simulink model "nn_fuel_control_5_10"  (R2021a)
settings: Solver=ode15s  StartTime=0.0  StopTime=T  MaxStep=.01  RelTol=1e-3
undefined symbols (not defined in the file): AF_sensor_tol, fault_time, fuel_inj_tol, kappa_tol, MAF_sensor_tol, pump_tol, tau_ww_tol
libraries: neural x57
(part 2 of 2)

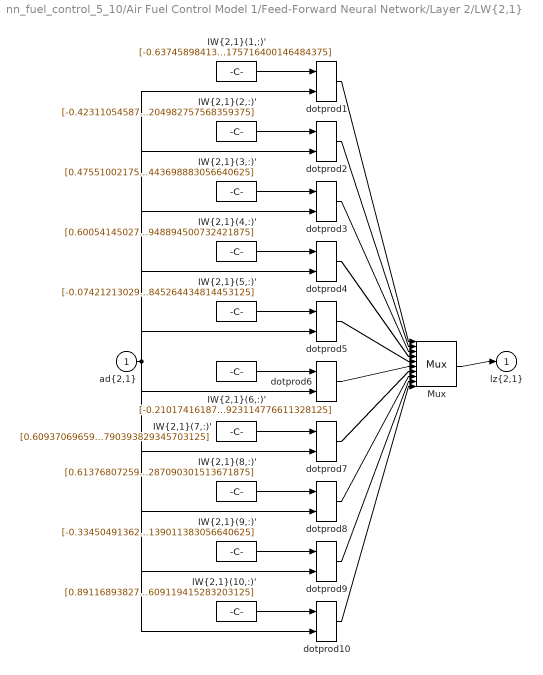
== system nn_fuel_control_5_10/Air Fuel Control Model 1/Feed-Forward Neural Network/Layer 2/LW{2,1} ==
  "ad{2,1}" : Inport  PortDimensions=10
      mask Display: e = 0.06;c1 = [120 230 180]/255;c2 = ([120 230 180]+0)/(256+128);c3 = ([120 230 180]+128)/(256+128);patch([0 1 1 0],[0 0 1 1],c1);patch([0 1 1 1-e 1-e 0+e],[0 0 1 1-e 0+e 0+e],c2);patch([0 0 1 1-e 0+e 0+e],[0 1 1 1-e 1-e 0+e],c3);plot([0 1 1 0 0],[0 0 1 1 0]);
  "IW{2,1}(1,:)'" : Constant  Value=[-0.637458984139413598057899434934370219707489013671875;0.8966217246671168705773879992193542420864105224609375;-0.0203090886026930927954481376218609511852264404296875;-0.412824398884275911569829986547119915485382080078125;-0.2423503469494130424521927125169895589351654052734375;0.9041152712576534522526117143570445477962493896484375;0.0771360103896812088208889690577052533626556396484375;-0.5024621550745056453024517395533621311187744140625;-0.2575893308760581756899910033098421990871429443359375;-0.6905985775161285200596239519654773175716400146484375]
      mask Display: e = 0.06;c1 = [120 150 230]/255;c2 = ([120 150 230]+0)/383;c3 = ([120 150 230]+128)/383;patch([0 1 1 0],[0 0 1 1],c1);patch([0 1 1 1-e 1-e 0+e],[0 0 1 1-e 0+e 0+e],c2);patch([0 0 1 1-e 0+e 0+e],[0 1 1 1-e 1-e 0+e],c3);plot([0 1 1 0 0],[0 0 1 1 0]);disp('weights');
  "IW{2,1}(10,:)'" : Constant  Value=[0.89116893827174614717279155229334719479084014892578125;-0.138771685053732329873099615724640898406505584716796875;0.360066357677085335797784182432224042713642120361328125;-0.486266631272339822089634253643453121185302734375;0.70490108854026178875074037932790815830230712890625;-0.96673858598125861352201582121779210865497589111328125;-0.206458691092018031820742862691986374557018280029296875;-0.96339598717867447330576169406413100659847259521484375;0.8351387726501771080478420117287896573543548583984375;0.2185868428207282665454158632201142609119415283203125]
      mask Display: e = 0.06;c1 = [120 150 230]/255;c2 = ([120 150 230]+0)/383;c3 = ([120 150 230]+128)/383;patch([0 1 1 0],[0 0 1 1],c1);patch([0 1 1 1-e 1-e 0+e],[0 0 1 1-e 0+e 0+e],c2);patch([0 0 1 1-e 0+e 0+e],[0 1 1 1-e 1-e 0+e],c3);plot([0 1 1 0 0],[0 0 1 1 0]);disp('weights');
  "IW{2,1}(2,:)'" : Constant  Value=[-0.423110545874279708744580830170889385044574737548828125;0.2368532384729105377818569877490517683327198028564453125;1.0125614808797680499452553704031743109226226806640625;0.991350908230053118330715733463875949382781982421875;0.5859879599201758271220796814304776489734649658203125;0.6228416385910036101591913393349386751651763916015625;0.66297446165075479829198457082384265959262847900390625;-0.68249454455804670072183171214419417083263397216796875;-0.2731411644690309170613318201503716409206390380859375;0.7259508101752485398350245304754935204982757568359375]
      mask Display: e = 0.06;c1 = [120 150 230]/255;c2 = ([120 150 230]+0)/383;c3 = ([120 150 230]+128)/383;patch([0 1 1 0],[0 0 1 1],c1);patch([0 1 1 1-e 1-e 0+e],[0 0 1 1-e 0+e 0+e],c2);patch([0 0 1 1-e 0+e 0+e],[0 1 1 1-e 1-e 0+e],c3);plot([0 1 1 0 0],[0 0 1 1 0]);disp('weights');
  "IW{2,1}(3,:)'" : Constant  Value=[0.47551002175782264291825640611932612955570220947265625;0.08086399994805872071257368816077359952032566070556640625;0.65153887054984982452054964596754871308803558349609375;-0.390853469357781424520226210006512701511383056640625;0.4244387850223023672668887229519896209239959716796875;0.69780646247800970360941619219374842941761016845703125;-0.422605255513745337037079252695548348128795623779296875;0.1356374397477954907298425268891151063144207000732421875;-0.799602102088680322111713394406251609325408935546875;0.3829313320921274854669036358245648443698883056640625]
      mask Display: e = 0.06;c1 = [120 150 230]/255;c2 = ([120 150 230]+0)/383;c3 = ([120 150 230]+128)/383;patch([0 1 1 0],[0 0 1 1],c1);patch([0 1 1 1-e 1-e 0+e],[0 0 1 1-e 0+e 0+e],c2);patch([0 0 1 1-e 0+e 0+e],[0 1 1 1-e 1-e 0+e],c3);plot([0 1 1 0 0],[0 0 1 1 0]);disp('weights');
  "IW{2,1}(4,:)'" : Constant  Value=[0.6005414502795767273113369810744188725948333740234375;11.4320674147867809011813733377493917942047119140625;0.421951948405398014063649725358118303120136260986328125;-0.037861256050832903241598614840768277645111083984375;-0.9949671896674103788171805717865936458110809326171875;-0.199969021175616656904594492516480386257171630859375;0.935316259593251597692642462789081037044525146484375;-0.94904454226816470363559119505225680768489837646484375;0.85670612621257102858862708671949803829193115234375;0.0801975162350963000079673292930237948894500732421875]
      mask Display: e = 0.06;c1 = [120 150 230]/255;c2 = ([120 150 230]+0)/383;c3 = ([120 150 230]+128)/383;patch([0 1 1 0],[0 0 1 1],c1);patch([0 1 1 1-e 1-e 0+e],[0 0 1 1-e 0+e 0+e],c2);patch([0 0 1 1-e 0+e 0+e],[0 1 1 1-e 1-e 0+e],c3);plot([0 1 1 0 0],[0 0 1 1 0]);disp('weights');
  "IW{2,1}(5,:)'" : Constant  Value=[-0.0742121302954270589680163539014756679534912109375;-0.1342580978786223067089622418279759585857391357421875;0.0915832479993226034054032425046898424625396728515625;-0.93787302986105913760184193961322307586669921875;-0.643811203007536025921808686689473688602447509765625;-0.116756066682536019385452163987793028354644775390625;-0.1435483736603855309255095562548376619815826416015625;-0.5110511184347534818783742593950591981410980224609375;-0.758544811567411603192567781661637127399444580078125;-0.398523306888638462197604894754476845264434814453125]
      mask Display: e = 0.06;c1 = [120 150 230]/255;c2 = ([120 150 230]+0)/383;c3 = ([120 150 230]+128)/383;patch([0 1 1 0],[0 0 1 1],c1);patch([0 1 1 1-e 1-e 0+e],[0 0 1 1-e 0+e 0+e],c2);patch([0 0 1 1-e 0+e 0+e],[0 1 1 1-e 1-e 0+e],c3);plot([0 1 1 0 0],[0 0 1 1 0]);disp('weights');
  "IW{2,1}(6,:)'" : Constant  Value=[-0.210174161874227660717906474019400775432586669921875;-0.3228525547071037227198075925116427242755889892578125;0.081467094240803117344285055878572165966033935546875;-0.223563749699733360642994739464484155178070068359375;0.55022795910762933857540701865218579769134521484375;0.1733910151474036265284439650713466107845306396484375;-0.4722076811425550690870522885234095156192779541015625;-0.7008127640379659961666902745491825044155120849609375;-0.7519677194670675302035078857443295419216156005859375;-0.134393425407410394001317399670369923114776611328125]
      mask Display: e = 0.06;c1 = [120 150 230]/255;c2 = ([120 150 230]+0)/383;c3 = ([120 150 230]+128)/383;patch([0 1 1 0],[0 0 1 1],c1);patch([0 1 1 1-e 1-e 0+e],[0 0 1 1-e 0+e 0+e],c2);patch([0 0 1 1-e 0+e 0+e],[0 1 1 1-e 1-e 0+e],c3);plot([0 1 1 0 0],[0 0 1 1 0]);disp('weights');
  "IW{2,1}(7,:)'" : Constant  Value=[0.6093706965999181601745249281520955264568328857421875;0.3953690665368394530077011950197629630565643310546875;0.084179609944530164877818378954543732106685638427734375;0.4749507737805398477348717278800904750823974609375;0.66685673515731735960798687301576137542724609375;0.478883610897159084363039482923340983688831329345703125;-0.1708217128254700956091483021737076342105865478515625;0.268209410222957078673289288417436182498931884765625;-0.97388905831939087676119015668518841266632080078125;-0.4246705658523748372346062751603312790393829345703125]
      mask Display: e = 0.06;c1 = [120 150 230]/255;c2 = ([120 150 230]+0)/383;c3 = ([120 150 230]+128)/383;patch([0 1 1 0],[0 0 1 1],c1);patch([0 1 1 1-e 1-e 0+e],[0 0 1 1-e 0+e 0+e],c2);patch([0 0 1 1-e 0+e 0+e],[0 1 1 1-e 1-e 0+e],c3);plot([0 1 1 0 0],[0 0 1 1 0]);disp('weights');
  "IW{2,1}(8,:)'" : Constant  Value=[0.6137680725996259578636227161041460931301116943359375;-1.191467660059975397501830229884944856166839599609375;0.7756199138359132216891111966106109321117401123046875;-0.837639262904835479872645009891130030155181884765625;0.89500835157132652142308870679698884487152099609375;-0.45248395209114200543609740634565241634845733642578125;0.241077681509801300396844681017682887613773345947265625;0.234555770444050681877712349887588061392307281494140625;-0.7503101997745991180721603086567483842372894287109375;0.690380892111544852696169982664287090301513671875]
      mask Display: e = 0.06;c1 = [120 150 230]/255;c2 = ([120 150 230]+0)/383;c3 = ([120 150 230]+128)/383;patch([0 1 1 0],[0 0 1 1],c1);patch([0 1 1 1-e 1-e 0+e],[0 0 1 1-e 0+e 0+e],c2);patch([0 0 1 1-e 0+e 0+e],[0 1 1 1-e 1-e 0+e],c3);plot([0 1 1 0 0],[0 0 1 1 0]);disp('weights');
  "IW{2,1}(9,:)'" : Constant  Value=[-0.3345049136284374835526023161946795880794525146484375;0.18594208697542580210892992909066379070281982421875;0.6455995939500607239125429259729571640491485595703125;-0.7707899293641851112823815128649584949016571044921875;-0.075594471798157147901520147570408880710601806640625;0.06163623848505039859446696937084197998046875;-0.213693913452614570047671804786659777164459228515625;-0.6393005766123474042927909977152012288570404052734375;-0.6056315881196070449732360430061817169189453125;-0.2241069216575370948163481443771161139011383056640625]
      mask Display: e = 0.06;c1 = [120 150 230]/255;c2 = ([120 150 230]+0)/383;c3 = ([120 150 230]+128)/383;patch([0 1 1 0],[0 0 1 1],c1);patch([0 1 1 1-e 1-e 0+e],[0 0 1 1-e 0+e 0+e],c2);patch([0 0 1 1-e 0+e 0+e],[0 1 1 1-e 1-e 0+e],c3);plot([0 1 1 0 0],[0 0 1 1 0]);disp('weights');
  Mux : Mux  Inputs=10
      mask Display: e = 0.06;c1 = [120 150 230]/255;c2 = ([120 150 230]+0)/383;c3 = ([120 150 230]+128)/383;patch([0 1 1 0],[0 0 1 1],c1);patch([0 1 1 1-e 1-e 0+e],[0 0 1 1-e 0+e 0+e],c2);patch([0 0 1 1-e 0+e 0+e],[0 1 1 1-e 1-e 0+e],c3);plot([0 1 1 0 0],[0 0 1 1 0]);disp('Mux');
  dotprod{1..10} (10 alike) : neural/Weight Functions/dotprod
  "lz{2,1}" : Outport
      mask Display: e = 0.06;c1 = [120 230 180]/255;c2 = ([120 230 180]+0)/(256+128);c3 = ([120 230 180]+128)/(256+128);patch([0 1 1 0],[0 0 1 1],c1);patch([0 1 1 1-e 1-e 0+e],[0 0 1 1-e 0+e 0+e],c2);patch([0 0 1 1-e 0+e 0+e],[0 1 1 1-e 1-e 0+e],c3);plot([0 1 1 0 0],[0 0 1 1 0]);
  wires:
  "IW{2,1}(1,:)'"/1 -> dotprod1/1
  "ad{2,1}"/1 -> dotprod1/2, dotprod2/2, dotprod3/2, dotprod4/2, dotprod5/2, dotprod6/2, dotprod7/2, dotprod8/2, dotprod9/2, dotprod10/2
  dotprod1/1 -> Mux/1
  "IW{2,1}(2,:)'"/1 -> dotprod2/1
  dotprod2/1 -> Mux/2
  "IW{2,1}(3,:)'"/1 -> dotprod3/1
  dotprod3/1 -> Mux/3
  "IW{2,1}(4,:)'"/1 -> dotprod4/1
  dotprod4/1 -> Mux/4
  "IW{2,1}(5,:)'"/1 -> dotprod5/1
  dotprod5/1 -> Mux/5
  "IW{2,1}(6,:)'"/1 -> dotprod6/1
  dotprod6/1 -> Mux/6
  "IW{2,1}(7,:)'"/1 -> dotprod7/1
  dotprod7/1 -> Mux/7
  "IW{2,1}(8,:)'"/1 -> dotprod8/1
  dotprod8/1 -> Mux/8
  "IW{2,1}(9,:)'"/1 -> dotprod9/1
  dotprod9/1 -> Mux/9
  "IW{2,1}(10,:)'"/1 -> dotprod10/1
  dotprod10/1 -> Mux/10
  Mux/1 -> "lz{2,1}"/1

== system nn_fuel_control_5_10/Air Fuel Control Model 1/Feed-Forward Neural Network/Layer 3/Delays 1 ==
  "p{3}" : Inport  PortDimensions=10
      mask Display: e = 0.06;c1 = [120 230 180]/255;c2 = ([120 230 180]+0)/(256+128);c3 = ([120 230 180]+128)/(256+128);patch([0 1 1 0],[0 0 1 1],c1);patch([0 1 1 1-e 1-e 0+e],[0 0 1 1-e 0+e 0+e],c2);patch([0 0 1 1-e 0+e 0+e],[0 1 1 1-e 1-e 0+e],c3);plot([0 1 1 0 0],[0 0 1 1 0]);
  mux : Mux  Inputs=1
      mask Display: e = 0.06;c1 = [120 150 230]/255;c2 = ([120 150 230]+0)/383;c3 = ([120 150 230]+128)/383;patch([0 1 1 0],[0 0 1 1],c1);patch([0 1 1 1-e 1-e 0+e],[0 0 1 1-e 0+e 0+e],c2);patch([0 0 1 1-e 0+e 0+e],[0 1 1 1-e 1-e 0+e],c3);plot([0 1 1 0 0],[0 0 1 1 0]);disp('Mux')
  "pd{3,2}" : Outport
      mask Display: e = 0.06;c1 = [120 230 180]/255;c2 = ([120 230 180]+0)/(256+128);c3 = ([120 230 180]+128)/(256+128);patch([0 1 1 0],[0 0 1 1],c1);patch([0 1 1 1-e 1-e 0+e],[0 0 1 1-e 0+e 0+e],c2);patch([0 0 1 1-e 0+e 0+e],[0 1 1 1-e 1-e 0+e],c3);plot([0 1 1 0 0],[0 0 1 1 0]);
  wires:
  "p{3}"/1 -> mux/1
  mux/1 -> "pd{3,2}"/1

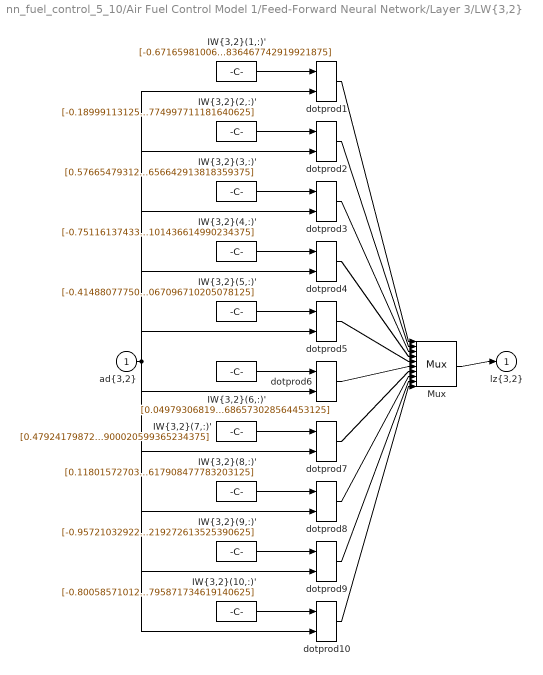
== system nn_fuel_control_5_10/Air Fuel Control Model 1/Feed-Forward Neural Network/Layer 3/LW{3,2} ==
  "ad{3,2}" : Inport  PortDimensions=10
      mask Display: e = 0.06;c1 = [120 230 180]/255;c2 = ([120 230 180]+0)/(256+128);c3 = ([120 230 180]+128)/(256+128);patch([0 1 1 0],[0 0 1 1],c1);patch([0 1 1 1-e 1-e 0+e],[0 0 1 1-e 0+e 0+e],c2);patch([0 0 1 1-e 0+e 0+e],[0 1 1 1-e 1-e 0+e],c3);plot([0 1 1 0 0],[0 0 1 1 0]);
  "IW{3,2}(1,:)'" : Constant  Value=[-0.6716598100666659743041009278385899960994720458984375;-0.09444487320076654091050016859298921190202236175537109375;0.30177109530501677880920397001318633556365966796875;-0.00726366674845616532019132449704557075165212154388427734375;-0.8447894134793438869479587083333171904087066650390625;0.413916207474557484857768940855748951435089111328125;-0.00906960978455077955484586738066354882903397083282470703125;0.383480564375462684711948213589494116604328155517578125;-0.816446131047855683249281355529092252254486083984375;-0.384774635045207424877133917107130400836467742919921875]
      mask Display: e = 0.06;c1 = [120 150 230]/255;c2 = ([120 150 230]+0)/383;c3 = ([120 150 230]+128)/383;patch([0 1 1 0],[0 0 1 1],c1);patch([0 1 1 1-e 1-e 0+e],[0 0 1 1-e 0+e 0+e],c2);patch([0 0 1 1-e 0+e 0+e],[0 1 1 1-e 1-e 0+e],c3);plot([0 1 1 0 0],[0 0 1 1 0]);disp('weights');
  "IW{3,2}(10,:)'" : Constant  Value=[-0.8005857101261424357829810105613432824611663818359375;-0.47743400890995635332814117646194063127040863037109375;-0.33193849760685478766930600613704882562160491943359375;0.32642190562985573532017724573961459100246429443359375;0.1192092790641339217216909673879854381084442138671875;0.623687154802713195067553897388279438018798828125;-0.2177505225475117878186637199178221635520458221435546875;0.69168924028525136105116644102963618934154510498046875;0.97190797419837959836286245263181626796722412109375;0.74205309722639400948906995836296118795871734619140625]
      mask Display: e = 0.06;c1 = [120 150 230]/255;c2 = ([120 150 230]+0)/383;c3 = ([120 150 230]+128)/383;patch([0 1 1 0],[0 0 1 1],c1);patch([0 1 1 1-e 1-e 0+e],[0 0 1 1-e 0+e 0+e],c2);patch([0 0 1 1-e 0+e 0+e],[0 1 1 1-e 1-e 0+e],c3);plot([0 1 1 0 0],[0 0 1 1 0]);disp('weights');
  "IW{3,2}(2,:)'" : Constant  Value=[-0.1899911312554338760349992298870347440242767333984375;0.234390586500404840553102303601917810738086700439453125;-0.156102985572256158786075275202165357768535614013671875;0.312828072064758544446050336773623712360858917236328125;-0.90271285913023380231834380538202822208404541015625;-0.378671814040422827218890233780257403850555419921875;-0.467712782650418545937753833641181699931621551513671875;-0.802890707313699270031293053762055933475494384765625;-0.2916201862903784469693846403970383107662200927734375;0.022119581342624261566243148990906774997711181640625]
      mask Display: e = 0.06;c1 = [120 150 230]/255;c2 = ([120 150 230]+0)/383;c3 = ([120 150 230]+128)/383;patch([0 1 1 0],[0 0 1 1],c1);patch([0 1 1 1-e 1-e 0+e],[0 0 1 1-e 0+e 0+e],c2);patch([0 0 1 1-e 0+e 0+e],[0 1 1 1-e 1-e 0+e],c3);plot([0 1 1 0 0],[0 0 1 1 0]);disp('weights');
  "IW{3,2}(3,:)'" : Constant  Value=[0.5766547931271384097584586925222538411617279052734375;-0.4621048397111515715351970357005484402179718017578125;-0.2677113161809201447027817266643978655338287353515625;-0.355326845647996325538997552939690649509429931640625;-0.550820658555060571615058506722562015056610107421875;-0.7951640335741243514888765275827609002590179443359375;-0.483849533444622892375264200381934642791748046875;-0.20635996968227399150919154635630548000335693359375;-0.8408541050908209246728119978797622025012969970703125;-0.64518665243028916478351675323210656642913818359375]
      mask Display: e = 0.06;c1 = [120 150 230]/255;c2 = ([120 150 230]+0)/383;c3 = ([120 150 230]+128)/383;patch([0 1 1 0],[0 0 1 1],c1);patch([0 1 1 1-e 1-e 0+e],[0 0 1 1-e 0+e 0+e],c2);patch([0 0 1 1-e 0+e 0+e],[0 1 1 1-e 1-e 0+e],c3);plot([0 1 1 0 0],[0 0 1 1 0]);disp('weights');
  "IW{3,2}(4,:)'" : Constant  Value=[-0.7511613743388598773975672884262166917324066162109375;-0.7073298684409738967815428622998297214508056640625;-0.1608146145951904470994264784167171455919742584228515625;-0.06609924042377292308092506800676346756517887115478515625;-0.3500290419633211858041477171354927122592926025390625;0.0806967197281041048739780308096669614315032958984375;0.214192490623146769568307945519336499273777008056640625;-0.65380194518047141105654418424819596111774444580078125;-0.953460508122269789765823588822968304157257080078125;0.9039040135586569046921567860408686101436614990234375]
      mask Display: e = 0.06;c1 = [120 150 230]/255;c2 = ([120 150 230]+0)/383;c3 = ([120 150 230]+128)/383;patch([0 1 1 0],[0 0 1 1],c1);patch([0 1 1 1-e 1-e 0+e],[0 0 1 1-e 0+e 0+e],c2);patch([0 0 1 1-e 0+e 0+e],[0 1 1 1-e 1-e 0+e],c3);plot([0 1 1 0 0],[0 0 1 1 0]);disp('weights');
  "IW{3,2}(5,:)'" : Constant  Value=[-0.4148807775058205304929970225202850997447967529296875;-0.8983006022029424997299429378472268581390380859375;-0.9871731677103785518312406566110439598560333251953125;-0.961342378972717792606772491126321256160736083984375;0.9734230145654325649928750863182358443737030029296875;-0.883253685041923919385453700670041143894195556640625;0.1002317592933905654462023449013940989971160888671875;-0.7961164864432699328489206891390495002269744873046875;0.7623659774831745838952201665961183607578277587890625;-0.0299654102361437413293288045679219067096710205078125]
      mask Display: e = 0.06;c1 = [120 150 230]/255;c2 = ([120 150 230]+0)/383;c3 = ([120 150 230]+128)/383;patch([0 1 1 0],[0 0 1 1],c1);patch([0 1 1 1-e 1-e 0+e],[0 0 1 1-e 0+e 0+e],c2);patch([0 0 1 1-e 0+e 0+e],[0 1 1 1-e 1-e 0+e],c3);plot([0 1 1 0 0],[0 0 1 1 0]);disp('weights');
  "IW{3,2}(6,:)'" : Constant  Value=[0.0497930681910487837882328676641918718814849853515625;-0.895592616306888800181695842184126377105712890625;0.70743332323692242891155501638422720134258270263671875;0.01217024604488731349960506378238278557546436786651611328125;-0.8087097508684788493837913847528398036956787109375;-0.2340048551736459980787685708492062985897064208984375;0.9150256608766491606132831293507479131221771240234375;0.0166745262836448353283014256476235459558665752410888671875;0.915985137420052719647856065421365201473236083984375;0.369222335473222973423190751418587751686573028564453125]
      mask Display: e = 0.06;c1 = [120 150 230]/255;c2 = ([120 150 230]+0)/383;c3 = ([120 150 230]+128)/383;patch([0 1 1 0],[0 0 1 1],c1);patch([0 1 1 1-e 1-e 0+e],[0 0 1 1-e 0+e 0+e],c2);patch([0 0 1 1-e 0+e 0+e],[0 1 1 1-e 1-e 0+e],c3);plot([0 1 1 0 0],[0 0 1 1 0]);disp('weights');
  "IW{3,2}(7,:)'" : Constant  Value=[0.479241798726635526151085286983288824558258056640625;-0.97240765217459024238877418611082248389720916748046875;-0.447624231578537756792712798414868302643299102783203125;-0.006737554878052109952335513298748992383480072021484375;-0.9089914321636864968922964180819690227508544921875;-0.825725336294859335595219818060286343097686767578125;0.68637707133362535483200872477027587592601776123046875;-0.499717536262347439279807304046698845922946929931640625;0.6827804263129746420446508636814542114734649658203125;-0.0258177275414916973517165388329885900020599365234375]
      mask Display: e = 0.06;c1 = [120 150 230]/255;c2 = ([120 150 230]+0)/383;c3 = ([120 150 230]+128)/383;patch([0 1 1 0],[0 0 1 1],c1);patch([0 1 1 1-e 1-e 0+e],[0 0 1 1-e 0+e 0+e],c2);patch([0 0 1 1-e 0+e 0+e],[0 1 1 1-e 1-e 0+e],c3);plot([0 1 1 0 0],[0 0 1 1 0]);disp('weights');
  "IW{3,2}(8,:)'" : Constant  Value=[0.1180157270398318747339772016857750713825225830078125;-0.739339538487907788066877401433885097503662109375;-0.49848365012323425649043429075391031801700592041015625;0.11760931477141882417480900357986683957278728485107421875;-0.972390077962221877072579445666633546352386474609375;0.280707542807327126155314545030705630779266357421875;0.29910352629640624133600113054853864014148712158203125;0.406498903852370585543241077175480313599109649658203125;0.1972911771665384339513593658921308815479278564453125;0.01986503978660032754266495658157509751617908477783203125]
      mask Display: e = 0.06;c1 = [120 150 230]/255;c2 = ([120 150 230]+0)/383;c3 = ([120 150 230]+128)/383;patch([0 1 1 0],[0 0 1 1],c1);patch([0 1 1 1-e 1-e 0+e],[0 0 1 1-e 0+e 0+e],c2);patch([0 0 1 1-e 0+e 0+e],[0 1 1 1-e 1-e 0+e],c3);plot([0 1 1 0 0],[0 0 1 1 0]);disp('weights');
  "IW{3,2}(9,:)'" : Constant  Value=[-0.9572103292253271167311368117225356400012969970703125;-0.0093351743505636353148702255566604435443878173828125;-0.7268216307528543307370227921637706458568572998046875;0.487521436827746013076279041342786513268947601318359375;-0.88712955957327022105118885519914329051971435546875;-0.502150672094246797172445440082810819149017333984375;-0.82513799604427673362039286075741983950138092041015625;0.15448203985870934129565057446598075330257415771484375;-0.182899890074335491618739979458041489124298095703125;0.42164247932195308976588421501219272613525390625]
      mask Display: e = 0.06;c1 = [120 150 230]/255;c2 = ([120 150 230]+0)/383;c3 = ([120 150 230]+128)/383;patch([0 1 1 0],[0 0 1 1],c1);patch([0 1 1 1-e 1-e 0+e],[0 0 1 1-e 0+e 0+e],c2);patch([0 0 1 1-e 0+e 0+e],[0 1 1 1-e 1-e 0+e],c3);plot([0 1 1 0 0],[0 0 1 1 0]);disp('weights');
  Mux : Mux  Inputs=10
      mask Display: e = 0.06;c1 = [120 150 230]/255;c2 = ([120 150 230]+0)/383;c3 = ([120 150 230]+128)/383;patch([0 1 1 0],[0 0 1 1],c1);patch([0 1 1 1-e 1-e 0+e],[0 0 1 1-e 0+e 0+e],c2);patch([0 0 1 1-e 0+e 0+e],[0 1 1 1-e 1-e 0+e],c3);plot([0 1 1 0 0],[0 0 1 1 0]);disp('Mux');
  dotprod{1..10} (10 alike) : neural/Weight Functions/dotprod
  "lz{3,2}" : Outport
      mask Display: e = 0.06;c1 = [120 230 180]/255;c2 = ([120 230 180]+0)/(256+128);c3 = ([120 230 180]+128)/(256+128);patch([0 1 1 0],[0 0 1 1],c1);patch([0 1 1 1-e 1-e 0+e],[0 0 1 1-e 0+e 0+e],c2);patch([0 0 1 1-e 0+e 0+e],[0 1 1 1-e 1-e 0+e],c3);plot([0 1 1 0 0],[0 0 1 1 0]);
  wires:
  "IW{3,2}(1,:)'"/1 -> dotprod1/1
  "ad{3,2}"/1 -> dotprod1/2, dotprod2/2, dotprod3/2, dotprod4/2, dotprod5/2, dotprod6/2, dotprod7/2, dotprod8/2, dotprod9/2, dotprod10/2
  dotprod1/1 -> Mux/1
  "IW{3,2}(2,:)'"/1 -> dotprod2/1
  dotprod2/1 -> Mux/2
  "IW{3,2}(3,:)'"/1 -> dotprod3/1
  dotprod3/1 -> Mux/3
  "IW{3,2}(4,:)'"/1 -> dotprod4/1
  dotprod4/1 -> Mux/4
  "IW{3,2}(5,:)'"/1 -> dotprod5/1
  dotprod5/1 -> Mux/5
  "IW{3,2}(6,:)'"/1 -> dotprod6/1
  dotprod6/1 -> Mux/6
  "IW{3,2}(7,:)'"/1 -> dotprod7/1
  dotprod7/1 -> Mux/7
  "IW{3,2}(8,:)'"/1 -> dotprod8/1
  dotprod8/1 -> Mux/8
  "IW{3,2}(9,:)'"/1 -> dotprod9/1
  dotprod9/1 -> Mux/9
  "IW{3,2}(10,:)'"/1 -> dotprod10/1
  dotprod10/1 -> Mux/10
  Mux/1 -> "lz{3,2}"/1

== system nn_fuel_control_5_10/Air Fuel Control Model 1/Feed-Forward Neural Network/Layer 4/Delays 1 ==
  "p{4}" : Inport  PortDimensions=10
      mask Display: e = 0.06;c1 = [120 230 180]/255;c2 = ([120 230 180]+0)/(256+128);c3 = ([120 230 180]+128)/(256+128);patch([0 1 1 0],[0 0 1 1],c1);patch([0 1 1 1-e 1-e 0+e],[0 0 1 1-e 0+e 0+e],c2);patch([0 0 1 1-e 0+e 0+e],[0 1 1 1-e 1-e 0+e],c3);plot([0 1 1 0 0],[0 0 1 1 0]);
  mux : Mux  Inputs=1
      mask Display: e = 0.06;c1 = [120 150 230]/255;c2 = ([120 150 230]+0)/383;c3 = ([120 150 230]+128)/383;patch([0 1 1 0],[0 0 1 1],c1);patch([0 1 1 1-e 1-e 0+e],[0 0 1 1-e 0+e 0+e],c2);patch([0 0 1 1-e 0+e 0+e],[0 1 1 1-e 1-e 0+e],c3);plot([0 1 1 0 0],[0 0 1 1 0]);disp('Mux')
  "pd{4,3}" : Outport
      mask Display: e = 0.06;c1 = [120 230 180]/255;c2 = ([120 230 180]+0)/(256+128);c3 = ([120 230 180]+128)/(256+128);patch([0 1 1 0],[0 0 1 1],c1);patch([0 1 1 1-e 1-e 0+e],[0 0 1 1-e 0+e 0+e],c2);patch([0 0 1 1-e 0+e 0+e],[0 1 1 1-e 1-e 0+e],c3);plot([0 1 1 0 0],[0 0 1 1 0]);
  wires:
  "p{4}"/1 -> mux/1
  mux/1 -> "pd{4,3}"/1

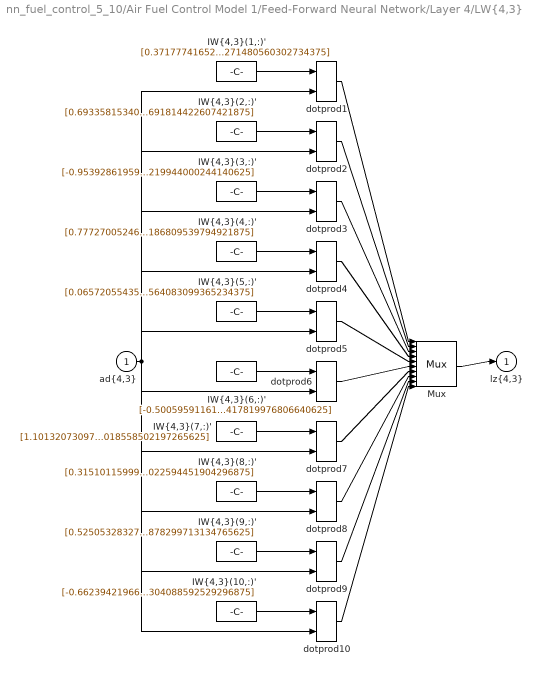
== system nn_fuel_control_5_10/Air Fuel Control Model 1/Feed-Forward Neural Network/Layer 4/LW{4,3} ==
  "ad{4,3}" : Inport  PortDimensions=10
      mask Display: e = 0.06;c1 = [120 230 180]/255;c2 = ([120 230 180]+0)/(256+128);c3 = ([120 230 180]+128)/(256+128);patch([0 1 1 0],[0 0 1 1],c1);patch([0 1 1 1-e 1-e 0+e],[0 0 1 1-e 0+e 0+e],c2);patch([0 0 1 1-e 0+e 0+e],[0 1 1 1-e 1-e 0+e],c3);plot([0 1 1 0 0],[0 0 1 1 0]);
  "IW{4,3}(1,:)'" : Constant  Value=[0.371777416527570958582060711705707944929599761962890625;-0.750769451156893641297074282192625105381011962890625;0.1692484502616806718577890933374874293804168701171875;-0.8167223528300053825290660824975930154323577880859375;0.359200076216012131880006563733331859111785888671875;-0.8895024378425639977052696849568746984004974365234375;-0.55543857115660788537070402526296675205230712890625;0.8812974391250623096283334234612993896007537841796875;-0.6803521057863932686160524099250324070453643798828125;-0.57314868500437421428017614744021557271480560302734375]
      mask Display: e = 0.06;c1 = [120 150 230]/255;c2 = ([120 150 230]+0)/383;c3 = ([120 150 230]+128)/383;patch([0 1 1 0],[0 0 1 1],c1);patch([0 1 1 1-e 1-e 0+e],[0 0 1 1-e 0+e 0+e],c2);patch([0 0 1 1-e 0+e 0+e],[0 1 1 1-e 1-e 0+e],c3);plot([0 1 1 0 0],[0 0 1 1 0]);disp('weights');
  "IW{4,3}(10,:)'" : Constant  Value=[-0.66239421966443778888589122288976795971393585205078125;0.538829260541769716752469321363605558872222900390625;0.9175095607354093463214894654811359941959381103515625;0.7595765677155486006455475944676436483860015869140625;0.75262175066824443803170652245171368122100830078125;1.0216703100890816013901485348469577729701995849609375;0.69096355864540004443341558726388029754161834716796875;-0.5396545202502538440825219367980025708675384521484375;-0.96005380573741394556464001652784645557403564453125;-0.76302222029962851745921170731890015304088592529296875]
      mask Display: e = 0.06;c1 = [120 150 230]/255;c2 = ([120 150 230]+0)/383;c3 = ([120 150 230]+128)/383;patch([0 1 1 0],[0 0 1 1],c1);patch([0 1 1 1-e 1-e 0+e],[0 0 1 1-e 0+e 0+e],c2);patch([0 0 1 1-e 0+e 0+e],[0 1 1 1-e 1-e 0+e],c3);plot([0 1 1 0 0],[0 0 1 1 0]);disp('weights');
  "IW{4,3}(2,:)'" : Constant  Value=[0.693358153408613731016885139979422092437744140625;0.748648558481644688100686835241504013538360595703125;0.364577299687717459875102576916106045246124267578125;0.76403922545622726669733992821420542895793914794921875;0.171578070945096694543963167234323918819427490234375;-0.15508816344271580955904710208415053784847259521484375;-0.25504814717701085324819132438278757035732269287109375;0.7350159561399618457500082513433881103992462158203125;-0.63728850904024458845498202208545990288257598876953125;0.70246056941893264546905584211344830691814422607421875]
      mask Display: e = 0.06;c1 = [120 150 230]/255;c2 = ([120 150 230]+0)/383;c3 = ([120 150 230]+128)/383;patch([0 1 1 0],[0 0 1 1],c1);patch([0 1 1 1-e 1-e 0+e],[0 0 1 1-e 0+e 0+e],c2);patch([0 0 1 1-e 0+e 0+e],[0 1 1 1-e 1-e 0+e],c3);plot([0 1 1 0 0],[0 0 1 1 0]);disp('weights');
  "IW{4,3}(3,:)'" : Constant  Value=[-0.9539286195965839265653585243853740394115447998046875;0.41286408504915517170275052194483578205108642578125;-0.305249109606310131681539132841862738132476806640625;0.830568443186014970791575251496396958827972412109375;-0.572829327914274433197761027258820831775665283203125;0.0023176300633893642810789970098994672298431396484375;0.9365350672959695810249058922636322677135467529296875;-0.92849168892259381635767567786388099193572998046875;-0.1049205075323824676303274827660061419010162353515625;-0.102548893764053961064064424135722219944000244140625]
      mask Display: e = 0.06;c1 = [120 150 230]/255;c2 = ([120 150 230]+0)/383;c3 = ([120 150 230]+128)/383;patch([0 1 1 0],[0 0 1 1],c1);patch([0 1 1 1-e 1-e 0+e],[0 0 1 1-e 0+e 0+e],c2);patch([0 0 1 1-e 0+e 0+e],[0 1 1 1-e 1-e 0+e],c3);plot([0 1 1 0 0],[0 0 1 1 0]);disp('weights');
  "IW{4,3}(4,:)'" : Constant  Value=[0.77727005246832725493533189364825375378131866455078125;0.439155932421952888145000315489596687257289886474609375;0.321693539016216778492207595263607800006866455078125;0.55984253870729350222035236583906225860118865966796875;0.7602682337948720725506746020982973277568817138671875;-0.14368490454010485191105317426263354718685150146484375;0.333719725231199582093921662817592732608318328857421875;0.51188221247608567399112189377774484455585479736328125;0.12485838815050953609642192532191984355449676513671875;0.85205658818599949722027986354078166186809539794921875]
      mask Display: e = 0.06;c1 = [120 150 230]/255;c2 = ([120 150 230]+0)/383;c3 = ([120 150 230]+128)/383;patch([0 1 1 0],[0 0 1 1],c1);patch([0 1 1 1-e 1-e 0+e],[0 0 1 1-e 0+e 0+e],c2);patch([0 0 1 1-e 0+e 0+e],[0 1 1 1-e 1-e 0+e],c3);plot([0 1 1 0 0],[0 0 1 1 0]);disp('weights');
  "IW{4,3}(5,:)'" : Constant  Value=[0.065720554359262772781136163757764734327793121337890625;-0.682418911141862150060433123144321143627166748046875;0.7729785581821724260720429811044596135616302490234375;-0.48339402285326349417715618983493186533451080322265625;-0.375739200911106241420611695502884685993194580078125;0.8263583879128686415782567564747296273708343505859375;0.58939348687387826952743807851220481097698211669921875;-0.2731442150571121718627409791224636137485504150390625;-0.55200084252227499259646492646425031125545501708984375;-0.62451709678290379113008157219155691564083099365234375]
      mask Display: e = 0.06;c1 = [120 150 230]/255;c2 = ([120 150 230]+0)/383;c3 = ([120 150 230]+128)/383;patch([0 1 1 0],[0 0 1 1],c1);patch([0 1 1 1-e 1-e 0+e],[0 0 1 1-e 0+e 0+e],c2);patch([0 0 1 1-e 0+e 0+e],[0 1 1 1-e 1-e 0+e],c3);plot([0 1 1 0 0],[0 0 1 1 0]);disp('weights');
  "IW{4,3}(6,:)'" : Constant  Value=[-0.5005959116130969110969317625858820974826812744140625;0.6376196795684443419105491557274945080280303955078125;0.73489591067990378547847285517491400241851806640625;0.6752296880622956631867737087304703891277313232421875;0.9484317972920646155898793949745595455169677734375;-0.2073882209696840117629790256614796817302703857421875;-0.0056272260834726584022291717701591551303863525390625;-0.36368541265910447890519208158366382122039794921875;0.1538505548184831983604681227006949484348297119140625;0.195791935445785103553362205275334417819976806640625]
      mask Display: e = 0.06;c1 = [120 150 230]/255;c2 = ([120 150 230]+0)/383;c3 = ([120 150 230]+128)/383;patch([0 1 1 0],[0 0 1 1],c1);patch([0 1 1 1-e 1-e 0+e],[0 0 1 1-e 0+e 0+e],c2);patch([0 0 1 1-e 0+e 0+e],[0 1 1 1-e 1-e 0+e],c3);plot([0 1 1 0 0],[0 0 1 1 0]);disp('weights');
  "IW{4,3}(7,:)'" : Constant  Value=[1.10132073097771776559739009826444089412689208984375;0.134859018158683507948580881929956376552581787109375;0.67669209867670421232332955696620047092437744140625;-581.465410711121194253792054951190948486328125;0.3973340542747367809539582594879902899265289306640625;-0.7557582299757739097145758933038450777530670166015625;0.4890033931306578818265506924944929778575897216796875;0.2443917239826218501530519233710947446525096893310546875;0.250510529596000453000925745072891004383563995361328125;0.52899307020386265865141695030615665018558502197265625]
      mask Display: e = 0.06;c1 = [120 150 230]/255;c2 = ([120 150 230]+0)/383;c3 = ([120 150 230]+128)/383;patch([0 1 1 0],[0 0 1 1],c1);patch([0 1 1 1-e 1-e 0+e],[0 0 1 1-e 0+e 0+e],c2);patch([0 0 1 1-e 0+e 0+e],[0 1 1 1-e 1-e 0+e],c3);plot([0 1 1 0 0],[0 0 1 1 0]);disp('weights');
  "IW{4,3}(8,:)'" : Constant  Value=[0.315101159996211410696531629582750611007213592529296875;0.131433110738516101267947533415281213819980621337890625;0.392838491111608067996030513313598930835723876953125;-0.68573955528896612943157151676132343709468841552734375;0.150463272728016850265930770547129213809967041015625;0.12168767033233239549527837652931339107453823089599609375;0.006034982597375948554230262743658386170864105224609375;1.0667707721596342285153014017851091921329498291015625;-0.1643001850726077128772573132664547301828861236572265625;0.335184674981723051967463788969325833022594451904296875]
      mask Display: e = 0.06;c1 = [120 150 230]/255;c2 = ([120 150 230]+0)/383;c3 = ([120 150 230]+128)/383;patch([0 1 1 0],[0 0 1 1],c1);patch([0 1 1 1-e 1-e 0+e],[0 0 1 1-e 0+e 0+e],c2);patch([0 0 1 1-e 0+e 0+e],[0 1 1 1-e 1-e 0+e],c3);plot([0 1 1 0 0],[0 0 1 1 0]);disp('weights');
  "IW{4,3}(9,:)'" : Constant  Value=[0.52505328327413292033298830574494786560535430908203125;0.4602525878961787331178356907912530004978179931640625;0.63320381749879661725799451232887804508209228515625;0.745529307542172947620429113158024847507476806640625;-0.70099819078384673076698163640685379505157470703125;-0.395370012291898331735495730754337273538112640380859375;-0.378580752216843396951162503683008253574371337890625;0.77086897035401091837769627090892754495143890380859375;-0.6506471456442908252171264393837191164493560791015625;0.83295933595360927004236373250023461878299713134765625]
      mask Display: e = 0.06;c1 = [120 150 230]/255;c2 = ([120 150 230]+0)/383;c3 = ([120 150 230]+128)/383;patch([0 1 1 0],[0 0 1 1],c1);patch([0 1 1 1-e 1-e 0+e],[0 0 1 1-e 0+e 0+e],c2);patch([0 0 1 1-e 0+e 0+e],[0 1 1 1-e 1-e 0+e],c3);plot([0 1 1 0 0],[0 0 1 1 0]);disp('weights');
  Mux : Mux  Inputs=10
      mask Display: e = 0.06;c1 = [120 150 230]/255;c2 = ([120 150 230]+0)/383;c3 = ([120 150 230]+128)/383;patch([0 1 1 0],[0 0 1 1],c1);patch([0 1 1 1-e 1-e 0+e],[0 0 1 1-e 0+e 0+e],c2);patch([0 0 1 1-e 0+e 0+e],[0 1 1 1-e 1-e 0+e],c3);plot([0 1 1 0 0],[0 0 1 1 0]);disp('Mux');
  dotprod{1..10} (10 alike) : neural/Weight Functions/dotprod
  "lz{4,3}" : Outport
      mask Display: e = 0.06;c1 = [120 230 180]/255;c2 = ([120 230 180]+0)/(256+128);c3 = ([120 230 180]+128)/(256+128);patch([0 1 1 0],[0 0 1 1],c1);patch([0 1 1 1-e 1-e 0+e],[0 0 1 1-e 0+e 0+e],c2);patch([0 0 1 1-e 0+e 0+e],[0 1 1 1-e 1-e 0+e],c3);plot([0 1 1 0 0],[0 0 1 1 0]);
  wires:
  "IW{4,3}(1,:)'"/1 -> dotprod1/1
  "ad{4,3}"/1 -> dotprod1/2, dotprod2/2, dotprod3/2, dotprod4/2, dotprod5/2, dotprod6/2, dotprod7/2, dotprod8/2, dotprod9/2, dotprod10/2
  dotprod1/1 -> Mux/1
  "IW{4,3}(2,:)'"/1 -> dotprod2/1
  dotprod2/1 -> Mux/2
  "IW{4,3}(3,:)'"/1 -> dotprod3/1
  dotprod3/1 -> Mux/3
  "IW{4,3}(4,:)'"/1 -> dotprod4/1
  dotprod4/1 -> Mux/4
  "IW{4,3}(5,:)'"/1 -> dotprod5/1
  dotprod5/1 -> Mux/5
  "IW{4,3}(6,:)'"/1 -> dotprod6/1
  dotprod6/1 -> Mux/6
  "IW{4,3}(7,:)'"/1 -> dotprod7/1
  dotprod7/1 -> Mux/7
  "IW{4,3}(8,:)'"/1 -> dotprod8/1
  dotprod8/1 -> Mux/8
  "IW{4,3}(9,:)'"/1 -> dotprod9/1
  dotprod9/1 -> Mux/9
  "IW{4,3}(10,:)'"/1 -> dotprod10/1
  dotprod10/1 -> Mux/10
  Mux/1 -> "lz{4,3}"/1

== system nn_fuel_control_5_10/Air Fuel Control Model 1/Feed-Forward Neural Network/Layer 5/Delays 1 ==
  "p{5}" : Inport  PortDimensions=10
      mask Display: e = 0.06;c1 = [120 230 180]/255;c2 = ([120 230 180]+0)/(256+128);c3 = ([120 230 180]+128)/(256+128);patch([0 1 1 0],[0 0 1 1],c1);patch([0 1 1 1-e 1-e 0+e],[0 0 1 1-e 0+e 0+e],c2);patch([0 0 1 1-e 0+e 0+e],[0 1 1 1-e 1-e 0+e],c3);plot([0 1 1 0 0],[0 0 1 1 0]);
  mux : Mux  Inputs=1
      mask Display: e = 0.06;c1 = [120 150 230]/255;c2 = ([120 150 230]+0)/383;c3 = ([120 150 230]+128)/383;patch([0 1 1 0],[0 0 1 1],c1);patch([0 1 1 1-e 1-e 0+e],[0 0 1 1-e 0+e 0+e],c2);patch([0 0 1 1-e 0+e 0+e],[0 1 1 1-e 1-e 0+e],c3);plot([0 1 1 0 0],[0 0 1 1 0]);disp('Mux')
  "pd{5,4}" : Outport
      mask Display: e = 0.06;c1 = [120 230 180]/255;c2 = ([120 230 180]+0)/(256+128);c3 = ([120 230 180]+128)/(256+128);patch([0 1 1 0],[0 0 1 1],c1);patch([0 1 1 1-e 1-e 0+e],[0 0 1 1-e 0+e 0+e],c2);patch([0 0 1 1-e 0+e 0+e],[0 1 1 1-e 1-e 0+e],c3);plot([0 1 1 0 0],[0 0 1 1 0]);
  wires:
  "p{5}"/1 -> mux/1
  mux/1 -> "pd{5,4}"/1

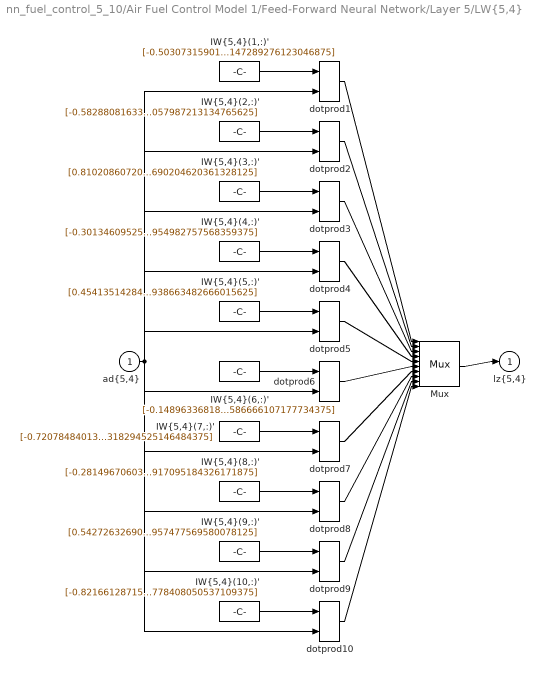
== system nn_fuel_control_5_10/Air Fuel Control Model 1/Feed-Forward Neural Network/Layer 5/LW{5,4} ==
  "ad{5,4}" : Inport  PortDimensions=10
      mask Display: e = 0.06;c1 = [120 230 180]/255;c2 = ([120 230 180]+0)/(256+128);c3 = ([120 230 180]+128)/(256+128);patch([0 1 1 0],[0 0 1 1],c1);patch([0 1 1 1-e 1-e 0+e],[0 0 1 1-e 0+e 0+e],c2);patch([0 0 1 1-e 0+e 0+e],[0 1 1 1-e 1-e 0+e],c3);plot([0 1 1 0 0],[0 0 1 1 0]);
  "IW{5,4}(1,:)'" : Constant  Value=[-0.50307315901935212298923261187155731022357940673828125;-0.157887772244862223391947964046266861259937286376953125;0.5727389957817485832691772884572856128215789794921875;-0.91729074349192984971779196712304838001728057861328125;0.74448917324784280591387641834444366395473480224609375;0.58775379603008293116772620123811066150665283203125;-734.4868977595375554301426745951175689697265625;0.70769139779057022021646616849466226994991302490234375;0.222210661253425201255851106907357461750507354736328125;-0.33481852066953077251554304893943481147289276123046875]
      mask Display: e = 0.06;c1 = [120 150 230]/255;c2 = ([120 150 230]+0)/383;c3 = ([120 150 230]+128)/383;patch([0 1 1 0],[0 0 1 1],c1);patch([0 1 1 1-e 1-e 0+e],[0 0 1 1-e 0+e 0+e],c2);patch([0 0 1 1-e 0+e 0+e],[0 1 1 1-e 1-e 0+e],c3);plot([0 1 1 0 0],[0 0 1 1 0]);disp('weights');
  "IW{5,4}(10,:)'" : Constant  Value=[-0.821661287156828290534349434892646968364715576171875;0.89076087711760332243926541195833124220371246337890625;0.0755930483345299553121776625630445778369903564453125;0.955385452003640889273583525209687650203704833984375;0.70556909697154257532503152106073684990406036376953125;0.8629777238059557209481909012538380920886993408203125;-0.448927536716850539288969912377069704234600067138671875;-0.51656134579686485697180842180387116968631744384765625;0.51320099944958708082509701853268779814243316650390625;-0.8269991497939022107033224529004655778408050537109375]
      mask Display: e = 0.06;c1 = [120 150 230]/255;c2 = ([120 150 230]+0)/383;c3 = ([120 150 230]+128)/383;patch([0 1 1 0],[0 0 1 1],c1);patch([0 1 1 1-e 1-e 0+e],[0 0 1 1-e 0+e 0+e],c2);patch([0 0 1 1-e 0+e 0+e],[0 1 1 1-e 1-e 0+e],c3);plot([0 1 1 0 0],[0 0 1 1 0]);disp('weights');
  "IW{5,4}(2,:)'" : Constant  Value=[-0.582880816332405071733546719769947230815887451171875;0.57856249760606004439722482857177965342998504638671875;0.4568197252672885344537689888966269791126251220703125;0.81436826248657456783774932773667387664318084716796875;0.64617343484303446654593017228762619197368621826171875;-0.9819703562352402048674093748559243977069854736328125;0.1575224552614240547399049319210462272167205810546875;0.1985729611386565507391566143269301392138004302978515625;-0.09981400185520199197508617316998424939811229705810546875;0.259095890901000436290502193514839746057987213134765625]
      mask Display: e = 0.06;c1 = [120 150 230]/255;c2 = ([120 150 230]+0)/383;c3 = ([120 150 230]+128)/383;patch([0 1 1 0],[0 0 1 1],c1);patch([0 1 1 1-e 1-e 0+e],[0 0 1 1-e 0+e 0+e],c2);patch([0 0 1 1-e 0+e 0+e],[0 1 1 1-e 1-e 0+e],c3);plot([0 1 1 0 0],[0 0 1 1 0]);disp('weights');
  "IW{5,4}(3,:)'" : Constant  Value=[0.8102086072069722977317951517761684954166412353515625;-0.67946031511730298202422773101716302335262298583984375;0.60809173232057833757835396681912243366241455078125;0.150526064013937588281777379961567930877208709716796875;0.78098137781740561980114989637513644993305206298828125;0.62331027873543831674396642483770847320556640625;0.225510942879522613413456610942375846207141876220703125;0.4199001787118061823633752283058129251003265380859375;-0.422930795475936205374267728984705172479152679443359375;0.046116837230647918233206183913353015668690204620361328125]
      mask Display: e = 0.06;c1 = [120 150 230]/255;c2 = ([120 150 230]+0)/383;c3 = ([120 150 230]+128)/383;patch([0 1 1 0],[0 0 1 1],c1);patch([0 1 1 1-e 1-e 0+e],[0 0 1 1-e 0+e 0+e],c2);patch([0 0 1 1-e 0+e 0+e],[0 1 1 1-e 1-e 0+e],c3);plot([0 1 1 0 0],[0 0 1 1 0]);disp('weights');
  "IW{5,4}(4,:)'" : Constant  Value=[-0.301346095252760959315452282680780626833438873291015625;0.67853521772802383171807605322101153433322906494140625;0.0475417753512583640684852070990018546581268310546875;0.92395204112239326388333893191884271800518035888671875;1.0050018339268687039833594099036417901515960693359375;0.3187208166570891787472419309779070317745208740234375;0.62309785119978811085417191861779429018497467041015625;0.212064763305431835949121932571870274841785430908203125;0.166045346543653049575794966585817746818065643310546875;-0.15465495433064402330813891239813528954982757568359375]
      mask Display: e = 0.06;c1 = [120 150 230]/255;c2 = ([120 150 230]+0)/383;c3 = ([120 150 230]+128)/383;patch([0 1 1 0],[0 0 1 1],c1);patch([0 1 1 1-e 1-e 0+e],[0 0 1 1-e 0+e 0+e],c2);patch([0 0 1 1-e 0+e 0+e],[0 1 1 1-e 1-e 0+e],c3);plot([0 1 1 0 0],[0 0 1 1 0]);disp('weights');
  "IW{5,4}(5,:)'" : Constant  Value=[0.4541351428464839301568645169027149677276611328125;-0.564781814809615756445282386266626417636871337890625;0.00206134840077698555660390411503612995147705078125;0.724253239706407203613025558297522366046905517578125;-0.7837575862468686427320108123240061104297637939453125;0.4753861655894062732130578297073952853679656982421875;-0.47521294355527299302366373012773692607879638671875;-0.37644206808346414305788130150176584720611572265625;-0.4679117307608431364229772952967323362827301025390625;-0.21202852056960441728961086482740938663482666015625]
      mask Display: e = 0.06;c1 = [120 150 230]/255;c2 = ([120 150 230]+0)/383;c3 = ([120 150 230]+128)/383;patch([0 1 1 0],[0 0 1 1],c1);patch([0 1 1 1-e 1-e 0+e],[0 0 1 1-e 0+e 0+e],c2);patch([0 0 1 1-e 0+e 0+e],[0 1 1 1-e 1-e 0+e],c3);plot([0 1 1 0 0],[0 0 1 1 0]);disp('weights');
  "IW{5,4}(6,:)'" : Constant  Value=[-0.1489633681886444460662488609159481711685657501220703125;0.60493719187068928366812770036631263792514801025390625;-0.451459498869969610979069329914636909961700439453125;0.49000305870791172058176243808702565729618072509765625;-0.481881293416142331142992816239711828529834747314453125;-0.833183537832906662146115195355378091335296630859375;-0.1972495610968268142659809427641448564827442169189453125;0.075382242306205993198631176710478030145168304443359375;-0.453829644255536346353352428195648826658725738525390625;-0.90859431836191839604310871436609886586666107177734375]
      mask Display: e = 0.06;c1 = [120 150 230]/255;c2 = ([120 150 230]+0)/383;c3 = ([120 150 230]+128)/383;patch([0 1 1 0],[0 0 1 1],c1);patch([0 1 1 1-e 1-e 0+e],[0 0 1 1-e 0+e 0+e],c2);patch([0 0 1 1-e 0+e 0+e],[0 1 1 1-e 1-e 0+e],c3);plot([0 1 1 0 0],[0 0 1 1 0]);disp('weights');
  "IW{5,4}(7,:)'" : Constant  Value=[-0.72078484013486132653270033188164234161376953125;-0.440129411875964660083582202787511050701141357421875;-0.083964219729971478756169744883663952350616455078125;0.187602726338339798051180196125642396509647369384765625;0.1893413861866903580288834518796647898852825164794921875;-0.1499363355269391906432474570465274155139923095703125;0.75554049437428350000089949389803223311901092529296875;0.94943138903241230952545492982608266174793243408203125;0.136645721474057235678145616475376300513744354248046875;0.6820236113431601410184157430194318294525146484375]
      mask Display: e = 0.06;c1 = [120 150 230]/255;c2 = ([120 150 230]+0)/383;c3 = ([120 150 230]+128)/383;patch([0 1 1 0],[0 0 1 1],c1);patch([0 1 1 1-e 1-e 0+e],[0 0 1 1-e 0+e 0+e],c2);patch([0 0 1 1-e 0+e 0+e],[0 1 1 1-e 1-e 0+e],c3);plot([0 1 1 0 0],[0 0 1 1 0]);disp('weights');
  "IW{5,4}(8,:)'" : Constant  Value=[-0.281496706031756527277565282929572276771068572998046875;0.48670246116335269537245267201797105371952056884765625;-0.8073318867623247019338350582984276115894317626953125;-0.69877823030923080782628176166326738893985748291015625;-0.59764443258303767692041219561360776424407958984375;0.656183564994172296991337134386412799358367919921875;-2037.265738881628976741922087967395782470703125;0.17081545090096372785382072834181599318981170654296875;-0.4352100641305940431635690401890315115451812744140625;1.0634320757483706199053585805813781917095184326171875]
      mask Display: e = 0.06;c1 = [120 150 230]/255;c2 = ([120 150 230]+0)/383;c3 = ([120 150 230]+128)/383;patch([0 1 1 0],[0 0 1 1],c1);patch([0 1 1 1-e 1-e 0+e],[0 0 1 1-e 0+e 0+e],c2);patch([0 0 1 1-e 0+e 0+e],[0 1 1 1-e 1-e 0+e],c3);plot([0 1 1 0 0],[0 0 1 1 0]);disp('weights');
  "IW{5,4}(9,:)'" : Constant  Value=[0.5427263269011108892669881242909468710422515869140625;0.184351109856324135716221235270495526492595672607421875;-0.5693096437000522147542369566508568823337554931640625;0.07058959467185281499990168185831862501800060272216796875;-0.877116993079829487811593935475684702396392822265625;-0.5956995554403896608874902085517533123493194580078125;0.1777893343421667327053370399880805052816867828369140625;0.43105096545809795660630925340228714048862457275390625;-0.64930318070306192179685922383214347064495086669921875;0.61449570957557420047834284559939987957477569580078125]
      mask Display: e = 0.06;c1 = [120 150 230]/255;c2 = ([120 150 230]+0)/383;c3 = ([120 150 230]+128)/383;patch([0 1 1 0],[0 0 1 1],c1);patch([0 1 1 1-e 1-e 0+e],[0 0 1 1-e 0+e 0+e],c2);patch([0 0 1 1-e 0+e 0+e],[0 1 1 1-e 1-e 0+e],c3);plot([0 1 1 0 0],[0 0 1 1 0]);disp('weights');
  Mux : Mux  Inputs=10
      mask Display: e = 0.06;c1 = [120 150 230]/255;c2 = ([120 150 230]+0)/383;c3 = ([120 150 230]+128)/383;patch([0 1 1 0],[0 0 1 1],c1);patch([0 1 1 1-e 1-e 0+e],[0 0 1 1-e 0+e 0+e],c2);patch([0 0 1 1-e 0+e 0+e],[0 1 1 1-e 1-e 0+e],c3);plot([0 1 1 0 0],[0 0 1 1 0]);disp('Mux');
  dotprod{1..10} (10 alike) : neural/Weight Functions/dotprod
  "lz{5,4}" : Outport
      mask Display: e = 0.06;c1 = [120 230 180]/255;c2 = ([120 230 180]+0)/(256+128);c3 = ([120 230 180]+128)/(256+128);patch([0 1 1 0],[0 0 1 1],c1);patch([0 1 1 1-e 1-e 0+e],[0 0 1 1-e 0+e 0+e],c2);patch([0 0 1 1-e 0+e 0+e],[0 1 1 1-e 1-e 0+e],c3);plot([0 1 1 0 0],[0 0 1 1 0]);
  wires:
  "IW{5,4}(1,:)'"/1 -> dotprod1/1
  "ad{5,4}"/1 -> dotprod1/2, dotprod2/2, dotprod3/2, dotprod4/2, dotprod5/2, dotprod6/2, dotprod7/2, dotprod8/2, dotprod9/2, dotprod10/2
  dotprod1/1 -> Mux/1
  "IW{5,4}(2,:)'"/1 -> dotprod2/1
  dotprod2/1 -> Mux/2
  "IW{5,4}(3,:)'"/1 -> dotprod3/1
  dotprod3/1 -> Mux/3
  "IW{5,4}(4,:)'"/1 -> dotprod4/1
  dotprod4/1 -> Mux/4
  "IW{5,4}(5,:)'"/1 -> dotprod5/1
  dotprod5/1 -> Mux/5
  "IW{5,4}(6,:)'"/1 -> dotprod6/1
  dotprod6/1 -> Mux/6
  "IW{5,4}(7,:)'"/1 -> dotprod7/1
  dotprod7/1 -> Mux/7
  "IW{5,4}(8,:)'"/1 -> dotprod8/1
  dotprod8/1 -> Mux/8
  "IW{5,4}(9,:)'"/1 -> dotprod9/1
  dotprod9/1 -> Mux/9
  "IW{5,4}(10,:)'"/1 -> dotprod10/1
  dotprod10/1 -> Mux/10
  Mux/1 -> "lz{5,4}"/1

== system nn_fuel_control_5_10/Air Fuel Control Model 1/Feed-Forward Neural Network/Layer 6/Delays 1 ==
  "p{6}" : Inport  PortDimensions=10
      mask Display: e = 0.06;c1 = [120 230 180]/255;c2 = ([120 230 180]+0)/(256+128);c3 = ([120 230 180]+128)/(256+128);patch([0 1 1 0],[0 0 1 1],c1);patch([0 1 1 1-e 1-e 0+e],[0 0 1 1-e 0+e 0+e],c2);patch([0 0 1 1-e 0+e 0+e],[0 1 1 1-e 1-e 0+e],c3);plot([0 1 1 0 0],[0 0 1 1 0]);
  mux : Mux  Inputs=1
      mask Display: e = 0.06;c1 = [120 150 230]/255;c2 = ([120 150 230]+0)/383;c3 = ([120 150 230]+128)/383;patch([0 1 1 0],[0 0 1 1],c1);patch([0 1 1 1-e 1-e 0+e],[0 0 1 1-e 0+e 0+e],c2);patch([0 0 1 1-e 0+e 0+e],[0 1 1 1-e 1-e 0+e],c3);plot([0 1 1 0 0],[0 0 1 1 0]);disp('Mux')
  "pd{6,5}" : Outport
      mask Display: e = 0.06;c1 = [120 230 180]/255;c2 = ([120 230 180]+0)/(256+128);c3 = ([120 230 180]+128)/(256+128);patch([0 1 1 0],[0 0 1 1],c1);patch([0 1 1 1-e 1-e 0+e],[0 0 1 1-e 0+e 0+e],c2);patch([0 0 1 1-e 0+e 0+e],[0 1 1 1-e 1-e 0+e],c3);plot([0 1 1 0 0],[0 0 1 1 0]);
  wires:
  "p{6}"/1 -> mux/1
  mux/1 -> "pd{6,5}"/1

== system nn_fuel_control_5_10/Air Fuel Control Model 1/Feed-Forward Neural Network/Layer 6/LW{6,5} ==
  "ad{6,5}" : Inport  PortDimensions=10
      mask Display: e = 0.06;c1 = [120 230 180]/255;c2 = ([120 230 180]+0)/(256+128);c3 = ([120 230 180]+128)/(256+128);patch([0 1 1 0],[0 0 1 1],c1);patch([0 1 1 1-e 1-e 0+e],[0 0 1 1-e 0+e 0+e],c2);patch([0 0 1 1-e 0+e 0+e],[0 1 1 1-e 1-e 0+e],c3);plot([0 1 1 0 0],[0 0 1 1 0]);
  "IW{6,5}(1,:)'" : Constant  Value=[1.51227223788125808567883723299019038677215576171875;0.88907328524462858609922477626241743564605712890625;0.83745028568932744494901498910621739923954010009765625;-0.60274725335459200525889400523738004267215728759765625;0.33465649647227824203810087055899202823638916015625;-0.82295846890516088922851167808403261005878448486328125;-1.0215175016615380965134818325168453156948089599609375;0.81375759478466935803453452535904943943023681640625;-1.2187849592755102268171185642131604254245758056640625;0.90698274702071601804931333390413783490657806396484375]
      mask Display: e = 0.06;c1 = [120 150 230]/255;c2 = ([120 150 230]+0)/383;c3 = ([120 150 230]+128)/383;patch([0 1 1 0],[0 0 1 1],c1);patch([0 1 1 1-e 1-e 0+e],[0 0 1 1-e 0+e 0+e],c2);patch([0 0 1 1-e 0+e 0+e],[0 1 1 1-e 1-e 0+e],c3);plot([0 1 1 0 0],[0 0 1 1 0]);disp('weights');
  Mux : Mux  Inputs=1
      mask Display: e = 0.06;c1 = [120 150 230]/255;c2 = ([120 150 230]+0)/383;c3 = ([120 150 230]+128)/383;patch([0 1 1 0],[0 0 1 1],c1);patch([0 1 1 1-e 1-e 0+e],[0 0 1 1-e 0+e 0+e],c2);patch([0 0 1 1-e 0+e 0+e],[0 1 1 1-e 1-e 0+e],c3);plot([0 1 1 0 0],[0 0 1 1 0]);disp('Mux');
  dotprod1 : neural/Weight Functions/dotprod
  "lz{6,5}" : Outport
      mask Display: e = 0.06;c1 = [120 230 180]/255;c2 = ([120 230 180]+0)/(256+128);c3 = ([120 230 180]+128)/(256+128);patch([0 1 1 0],[0 0 1 1],c1);patch([0 1 1 1-e 1-e 0+e],[0 0 1 1-e 0+e 0+e],c2);patch([0 0 1 1-e 0+e 0+e],[0 1 1 1-e 1-e 0+e],c3);plot([0 1 1 0 0],[0 0 1 1 0]);
  wires:
  "IW{6,5}(1,:)'"/1 -> dotprod1/1
  "ad{6,5}"/1 -> dotprod1/2
  dotprod1/1 -> Mux/1
  Mux/1 -> "lz{6,5}"/1
